simulink model "validation_and_interpretation"  (R2024a)
settings: Solver=VariableStepAuto  StartTime=0.0  StopTime=66  RelTol=1e-3
undefined symbols (not defined in the file): C, R
settings Model: Creator=osoko  LastModifiedBy=osoko

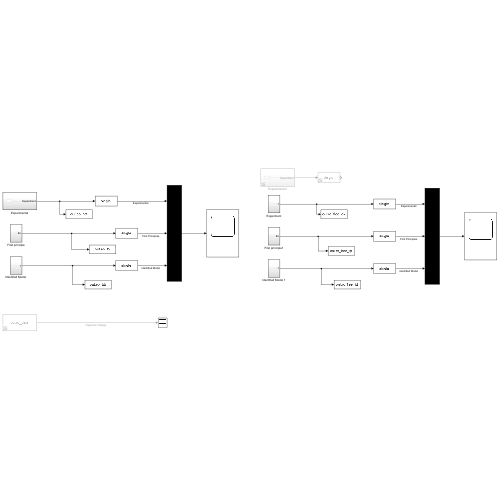
[thumbnail: Simulink's stored preview of the top-level diagram]
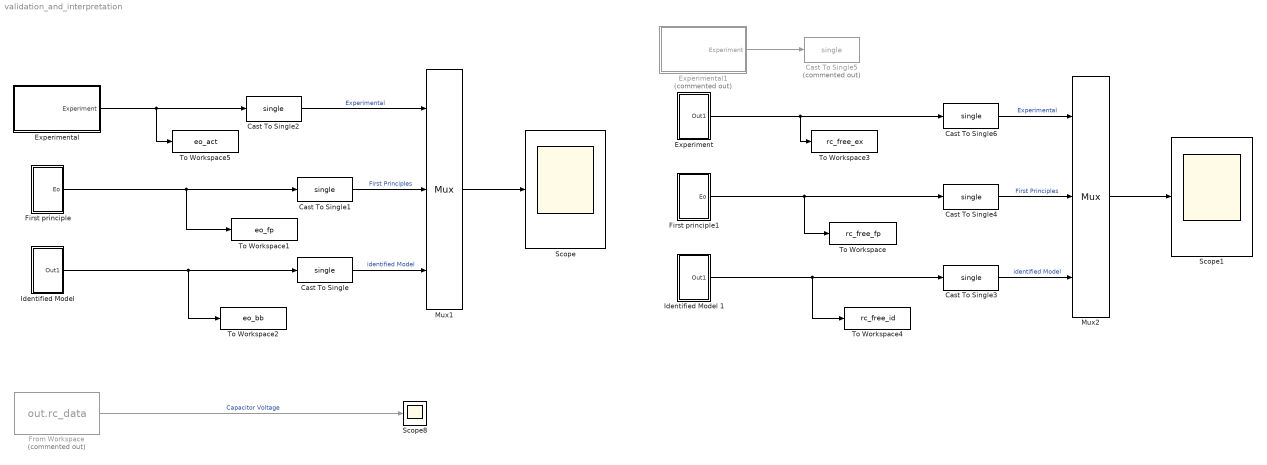
== system validation_and_interpretation ==
  Cast To Single{,1..4,6} (6 alike) : DataTypeConversion  OutDataTypeStr=single  SaturateOnIntegerOverflow=off  RndMeth=Floor
  Cast To Single5 : DataTypeConversion  Commented=on  OutDataTypeStr=single  SaturateOnIntegerOverflow=off  RndMeth=Floor
  Experiment : Subsystem
  Experimental : Subsystem
  Experimental1 : Subsystem  Commented=on
  First principle : Subsystem
  First principle1 : Subsystem
  From Workspace : FromWorkspace  Commented=on  VariableName=out.rc_data  OutDataTypeStr=double
  "Identified Model " : Subsystem
  Identified Model 1 : Subsystem
  Mux1 : Mux  Inputs=3
  Mux2 : Mux  Inputs=3
  Scope : Scope
  Scope1 : Scope
  Scope8 : Scope
  To Workspace : ToWorkspace  VariableName=rc_free_fp  SaveFormat=Structure With Time  SampleTime=-1
  To Workspace1 : ToWorkspace  VariableName=eo_fp  SaveFormat=Structure With Time  SampleTime=-1
  To Workspace2 : ToWorkspace  VariableName=eo_bb  SaveFormat=Structure With Time  SampleTime=-1
  To Workspace3 : ToWorkspace  VariableName=rc_free_ex  SaveFormat=Structure With Time  SampleTime=-1
  To Workspace4 : ToWorkspace  VariableName=rc_free_id  SaveFormat=Structure With Time  SampleTime=-1
  To Workspace5 : ToWorkspace  VariableName=eo_act  SaveFormat=Structure With Time  SampleTime=-1
  wires:
  "Identified Model "/1(Out1) -> Cast To Single/1, To Workspace2/1
  First principle/1(Eo) -> Cast To Single1/1, To Workspace1/1
  Experimental/1(Experiment) -> To Workspace5/1, Cast To Single2/1
  Mux1/1 -> Scope/1
  Cast To Single/1 -> Mux1/3  "identified Model"
  Cast To Single1/1 -> Mux1/2  "First Principles"
  From Workspace/1 -> Scope8/1  "Capacitor Voltage"
  Cast To Single2/1 -> Mux1/1  "Experimental"
  Mux2/1 -> Scope1/1
  Cast To Single3/1 -> Mux2/3  "identified Model"
  Cast To Single4/1 -> Mux2/2  "First Principles"
  First principle1/1(Eo) -> To Workspace/1, Cast To Single4/1
  Identified Model 1/1(Out1) -> To Workspace4/1, Cast To Single3/1
  Experiment/1(Out1) -> To Workspace3/1, Cast To Single6/1
  Experimental1/1(Experiment) -> Cast To Single5/1
  Cast To Single6/1 -> Mux2/1  "Experimental"

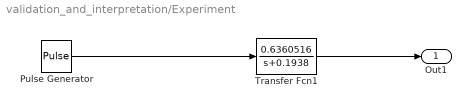
== system validation_and_interpretation/Experiment ==
  Pulse Generator : DiscretePulseGenerator  PulseType=Time based  Period=50  PulseWidth=63  PhaseDelay=18
  Transfer Fcn1 : TransferFcn  Numerator=[0.6360516]  Denominator=[1 0.1938]  ParameterTunability=Optimized
  Out1 : Outport
  wires:
  Transfer Fcn1/1 -> Out1/1
  Pulse Generator/1 -> Transfer Fcn1/1

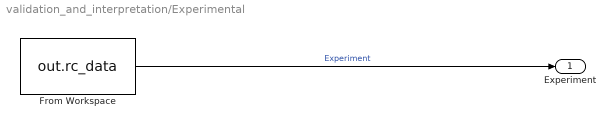
== system validation_and_interpretation/Experimental ==
  From Workspace : FromWorkspace  VariableName=out.rc_data  OutDataTypeStr=double
  Experiment : Outport
  wires:
  From Workspace/1 -> Experiment/1  "Experiment"

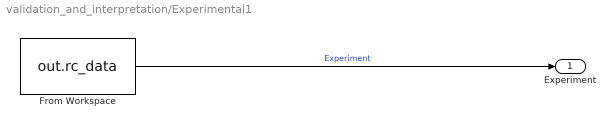
== system validation_and_interpretation/Experimental1 ==
  From Workspace : FromWorkspace  VariableName=out.rc_data  OutDataTypeStr=double
  Experiment : Outport
  wires:
  From Workspace/1 -> Experiment/1  "Experiment"

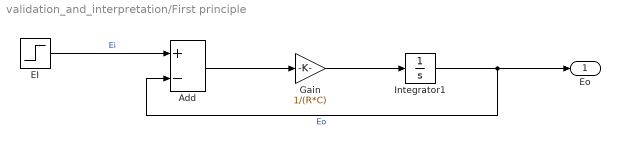
== system validation_and_interpretation/First principle ==
  Add : Sum  Inputs=+-  AccumDataTypeStr=single
  EI : Step  Time=0  After=3.28  OutDataTypeStr=single  SampleTime=0
  Gain : Gain  Gain=1/(R*C)  OutDataTypeStr=Inherit: Same as input
  Integrator1 : Integrator
  Eo : Outport
  wires:
  Integrator1/1 -> Eo/1, Add/2  "Eo"
  Add/1 -> Gain/1
  EI/1 -> Add/1  "Ei"
  Gain/1 -> Integrator1/1

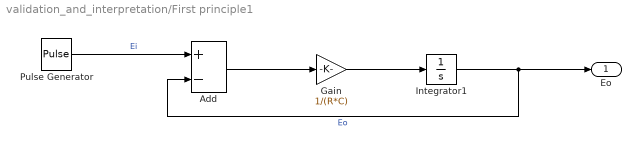
== system validation_and_interpretation/First principle1 ==
  Add : Sum  Inputs=+-  AccumDataTypeStr=single
  Gain : Gain  Gain=1/(R*C)  OutDataTypeStr=Inherit: Same as input
  Integrator1 : Integrator
  Pulse Generator : DiscretePulseGenerator  PulseType=Time based  Amplitude=3.3  Period=50  PulseWidth=63  PhaseDelay=18
  Eo : Outport
  wires:
  Integrator1/1 -> Eo/1, Add/2  "Eo"
  Add/1 -> Gain/1
  Pulse Generator/1 -> Add/1  "Ei"
  Gain/1 -> Integrator1/1

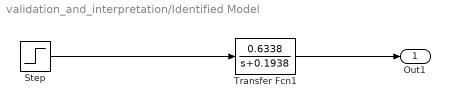
== system validation_and_interpretation/Identified Model  ==
  Step : Step  Time=0  SampleTime=0
  Transfer Fcn1 : TransferFcn  Numerator=[0.6338]  Denominator=[1 0.1938]  ParameterTunability=Optimized
  Out1 : Outport
  wires:
  Transfer Fcn1/1 -> Out1/1
  Step/1 -> Transfer Fcn1/1

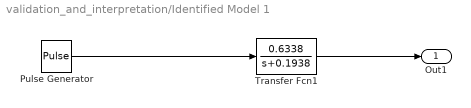
== system validation_and_interpretation/Identified Model 1 ==
  Pulse Generator : DiscretePulseGenerator  PulseType=Time based  Period=50  PulseWidth=63  PhaseDelay=18
  Transfer Fcn1 : TransferFcn  Numerator=[0.6338]  Denominator=[1 0.1938]  ParameterTunability=Optimized
  Out1 : Outport
  wires:
  Transfer Fcn1/1 -> Out1/1
  Pulse Generator/1 -> Transfer Fcn1/1
